simulink model "closedloop_DE_B"  (R2017a)
settings: Solver=FixedStepDiscrete  StartTime=0.0  StopTime=Tf  FixedStep=Ts  RelTol=1e-3  EnableMultiTasking=on
values from neighbouring files (symbols this model uses):
  Ts = t(2)-t(1)    [check_filter.m]    (also in closedloop_driver.m = 0.1; openloop_driver.m = 0.1; wheel_parameters.m = 0.05)
libraries: simulink x4
settings Model: Creator=throne  LastModifiedBy=localmgr
settings DataIOCC: LimitDataPoints=on  SaveFormat=Array
settings OptimizationCC: ExpressionDepthLimit=2147483647  InitFltsAndDblsToZero=on  LifeSpan=inf
settings DebuggingCC: UnderspecifiedInitializationDetection=Classic  MergeDetectMultiDrivingBlocksExec=none  SolverPrmCheckMsg=warning  StateNameClashWarn=warning  SFUnexpectedBacktrackingDiag=warning  SFNoUnconditionalDefaultTransitionDiag=warning  SFExecutionAtInitializationDiag=none
settings HardwareCC: ProdBitPerPointer=32  ProdBitPerSizeT=32  ProdBitPerPtrDiffT=32  ProdLargestAtomicFloat=None  ProdIntDivRoundTo=Undefined  ProdEndianess=Unspecified  ProdWordSize=32  ProdHWDeviceType=32-bit Generic
settings ModelReferenceCC: PropagateSignalLabelsOutOfModel=off
settings GRTTargetCC: TargetLangStandard=C89/C90 (ANSI)  GeneratePreprocessorConditionals=Disable all  CombineOutputUpdateFcns=off  GRTInterface=on
settings ConfigComp: CovMetricSettings=dw  CovHtmlReporting=on  CovSaveCumulativeToWorkspaceVar=on  CovSaveSingleToWorkspaceVar=on  CovExternalEMLEnable=off

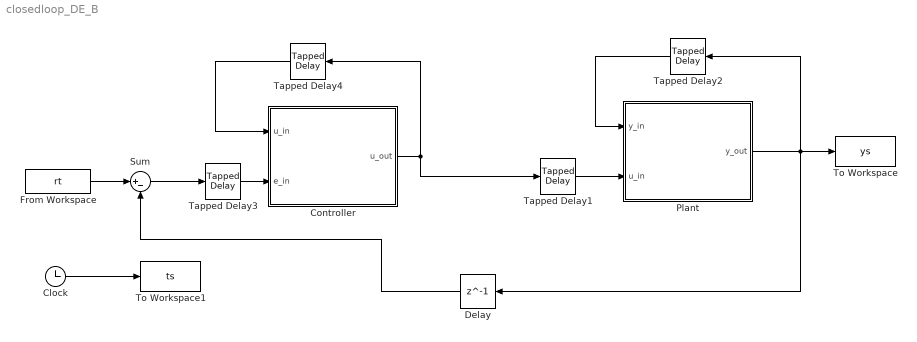
== system closedloop_DE_B ==
  " Controller" : MATLAB Function  TreatAsAtomicUnit=on
  " Plant" : MATLAB Function  TreatAsAtomicUnit=on
  Clock : Clock
  Delay : Delay  DelayLength=1  InitialCondition=0
  From Workspace : FromWorkspace  VariableName=rt  SampleTime=0
  Sum : Sum  Inputs=|+-
  Tapped Delay1 : simulink/Discrete/Tapped Delay  vinit=0.0  samptime=Ts  NumDelays=1  DelayOrder=Newest  includeCurrent=on
  Tapped Delay2 : simulink/Discrete/Tapped Delay  vinit=0.0  samptime=-1  NumDelays=1  DelayOrder=Newest  includeCurrent=on
  Tapped Delay3 : simulink/Discrete/Tapped Delay  vinit=0.0  samptime=Ts  NumDelays=1  DelayOrder=Newest  includeCurrent=on
  Tapped Delay4 : simulink/Discrete/Tapped Delay  vinit=0.0  samptime=-1  NumDelays=1  DelayOrder=Newest  includeCurrent=on
  To Workspace : ToWorkspace  VariableName=ys  SampleTime=-1
  To Workspace1 : ToWorkspace  VariableName=ts  SampleTime=Ts
  wires:
  Clock/1 -> To Workspace1/1
  Tapped Delay2/1 -> " Plant"/1(y_in)
  Tapped Delay1/1 -> " Plant"/2(u_in)
  " Plant"/1(y_out) -> Delay/1, To Workspace/1, Tapped Delay2/1
  " Controller"/1(u_out) -> Tapped Delay1/1, Tapped Delay4/1
  Tapped Delay4/1 -> " Controller"/1(u_in)
  Tapped Delay3/1 -> " Controller"/2(e_in)
  From Workspace/1 -> Sum/1
  Sum/1 -> Tapped Delay3/1
  Delay/1 -> Sum/2

== matlab function closedloop_DE_B/ Controller ==
  data: u_in input size=[1 2]; e_in input size=[1 2]; u_out output
function u_out  = fcn(u_in, e_in)
% This block supports the Embedded MATLAB subset.
% See the help menu for details. 
  u_out = u_in(2)+0.115*e_in(1) - 0.062905*e_in(2);

== matlab function closedloop_DE_B/ Plant ==
  data: y_in input size=[1 2]; u_in input size=[1 2]; y_out output
function y_out  = fcn(y_in, u_in)
% This block supports the Embedded MATLAB subset.
% See the help menu for details. 
  y_out = 0.8*y_in(2)+u_in(1) - 0.2 * u_in(2);
